simulink subsystem "actuators"  (R2022b)
settings: Solver=VariableStepAuto  StartTime=0.0  StopTime=10.0  RelTol=1e-3
undefined symbols (not defined in the file or in its folder): magnetorquers, thruster
libraries: matrix_library x5
settings Model: Creator=brent  LastModifiedBy=robertopistonenascone

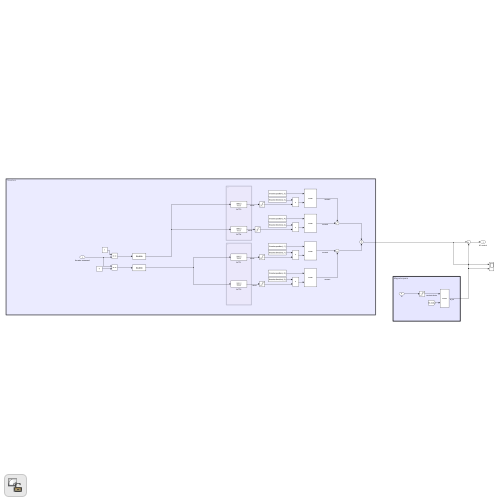
[thumbnail: Simulink's stored preview of the top-level diagram]
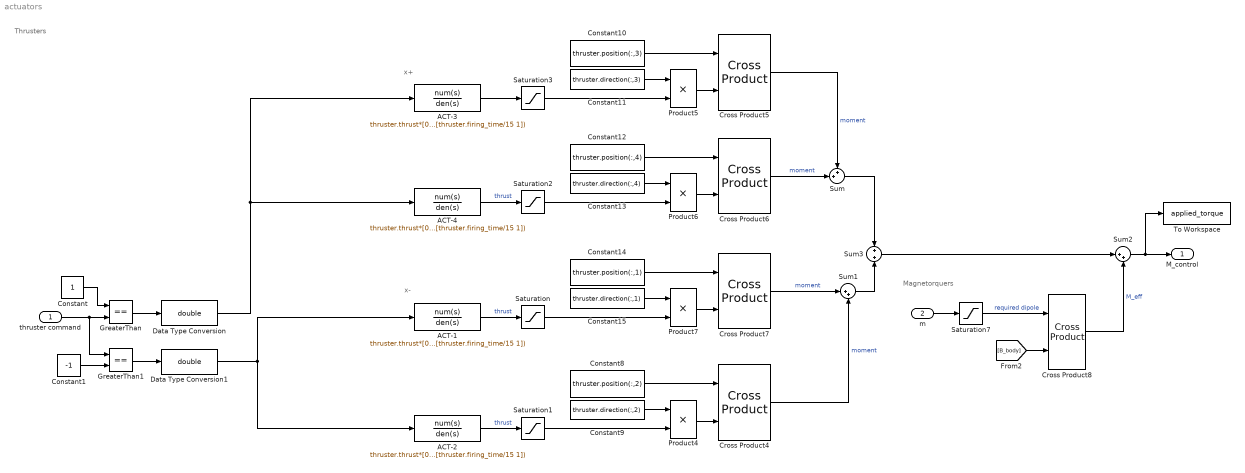
== system actuators ==
  note: Thrusters
  note: Magnetorquers
  note: x+
  note: x-
  thruster command : Inport
  m : Inport  Port=2
  ACT-{1..4} (4 alike) : TransferFcn  Numerator=thruster.thrust*[0.008 1]  Denominator=conv([(thruster.firing_time/15) 1],[thruster.firing_time/15 1])
  Constant : Constant
  Constant1 : Constant  Value=-1
  Constant10 : Constant  Value=thruster.position(:,3)
  Constant11 : Constant  Value=thruster.direction(:,3)
  Constant12 : Constant  Value=thruster.position(:,4)
  Constant13 : Constant  Value=thruster.direction(:,4)
  Constant14 : Constant  Value=thruster.position(:,1)
  Constant15 : Constant  Value=thruster.direction(:,1)
  Constant8 : Constant  Value=thruster.position(:,2)
  Constant9 : Constant  Value=thruster.direction(:,2)
  Cross Product{4..8} (5 alike) : matrix_library/Cross Product
  Data Type Conversion : DataTypeConversion  OutDataTypeStr=double  SaturateOnIntegerOverflow=off  RndMeth=Floor
  Data Type Conversion1 : DataTypeConversion  OutDataTypeStr=double  SaturateOnIntegerOverflow=off  RndMeth=Floor
  GreaterThan : RelationalOperator  Operator===  OutDataTypeStr=boolean  RndMeth=Simplest  InputSameDT=off
  GreaterThan1 : RelationalOperator  Operator===  OutDataTypeStr=boolean  RndMeth=Simplest  InputSameDT=off
  Product{4..7} (4 alike) : Product
  Saturation{,1..3} (4 alike) : Saturate  UpperLimit=inf  LowerLimit=0
  Saturation7 : Saturate  UpperLimit=magnetorquers.dipole  LowerLimit=-magnetorquers.dipole
  Sum : Sum  Inputs=++|
  Sum1 : Sum  Inputs=|++
  Sum2 : Sum  Inputs=|++
  Sum3 : Sum  Inputs=+|+
  To Workspace : ToWorkspace  VariableName=applied_torque  SampleTime=-1
  M_control : Outport
  wires:
  ACT-2/1 -> Saturation1/1  "thrust"
  Cross Product4/1 -> Sum1/2  "moment"
  Constant8/1 -> Cross Product4/1
  Constant9/1 -> Product4/1
  Cross Product5/1 -> Sum/1  "moment"
  Product5/1 -> Cross Product5/2
  Constant10/1 -> Cross Product5/1
  Constant11/1 -> Product5/1
  Constant13/1 -> Product6/1
  Constant12/1 -> Cross Product6/1
  Cross Product6/1 -> Sum/2  "moment"
  ACT-4/1 -> Saturation2/1  "thrust"
  Product6/1 -> Cross Product6/2
  ACT-1/1 -> Saturation/1  "thrust"
  Constant15/1 -> Product7/1
  Cross Product7/1 -> Sum1/1  "moment"
  Product4/1 -> Cross Product4/2
  Constant14/1 -> Cross Product7/1
  Product7/1 -> Cross Product7/2
  Saturation1/1 -> Product4/2
  Saturation3/1 -> Product5/2
  Saturation2/1 -> Product6/2
  Saturation/1 -> Product7/2
  [B_body] -> Cross Product8/2
  Saturation7/1 -> Cross Product8/1  "required dipole"
  m/1 -> Saturation7/1
  Sum1/1 -> Sum3/2
  Sum/1 -> Sum3/1
  Sum3/1 -> Sum2/1
  Cross Product8/1 -> Sum2/2  "M_eff"
  Constant/1 -> GreaterThan/1
  GreaterThan/1 -> Data Type Conversion/1
  Constant1/1 -> GreaterThan1/2
  GreaterThan1/1 -> Data Type Conversion1/1
  Data Type Conversion/1 -> ACT-4/1, ACT-3/1
  Data Type Conversion1/1 -> ACT-1/1, ACT-2/1
  ACT-3/1 -> Saturation3/1
  Sum2/1 -> M_control/1, To Workspace/1
  thruster command/1 -> GreaterThan/2, GreaterThan1/1
